simulink model "VOO"  (R2022a)
settings: Solver=FixedStepAuto  StartTime=0.0  StopTime=5  FixedStep=1e-3  RelTol=1e-3  EnableMultiTasking=on
undefined symbols (not defined in the file): D10, D11, D12, D2, D5, D8, D9, PTA0, PTA2, PTB9, PTC4, PTD0, PTD2, PTD3
libraries: frdmk64flib x8
settings Model: ExtModeTrigDuration=5  Creator=tygre  LastModifiedBy=tygre
settings OptimizationCC: EnhancedBackFolding=on  PassReuseOutputArgsAs=Individual arguments  ZeroExternalMemoryAtStartup=off  ZeroInternalMemoryAtStartup=off  MaxStackSize=64  OptimizeBlockOrder=speed  DifferentSizesBufferReuse=on  OptimizationCustomize=off  EfficientTunableParamExpr=on
settings DebuggingCC: ParameterTunabilityLossMsg=error
settings HardwareCC: ProdBitPerPointer=32  ProdBitPerSizeT=32  ProdBitPerPtrDiffT=32  ProdLargestAtomicInteger=Long  ProdLargestAtomicFloat=Double  ProdWordSize=32  ProdHWDeviceType=ARM Compatible->ARM Cortex
settings SFSimCC: MATLABDynamicMemAlloc=off
settings RTWCC: SystemTargetFile=ert.tlc  HardwareBoard=NXP FRDM-K64F  TLCOptions="-aInlineSetEventsForThisBaseRateFcn=TLC_FALSE -aSuppressMultiTaskScheduler=TLC_FALSE  -aRateBasedStepFcn=0"  TemplateMakefile=ert_default_tmf  Toolchain=GNU Tools for ARM Embedded Processors
settings CodeAppCC: ForceParamTrailComments=on  IgnoreCustomStorageClasses=off  OperatorAnnotations=on  SimulinkDataObjDesc=on  SFDataObjDesc=on  InsertBlockDesc=on
settings ERTTargetCC: ExtModeTransport=4  ExtModeMexFile=sendToCommService

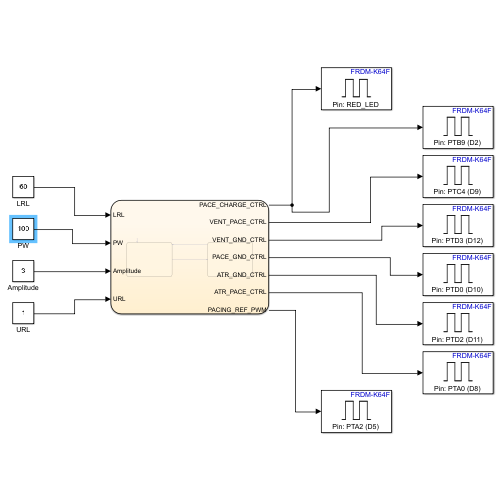
[thumbnail: Simulink's stored preview of the top-level diagram]
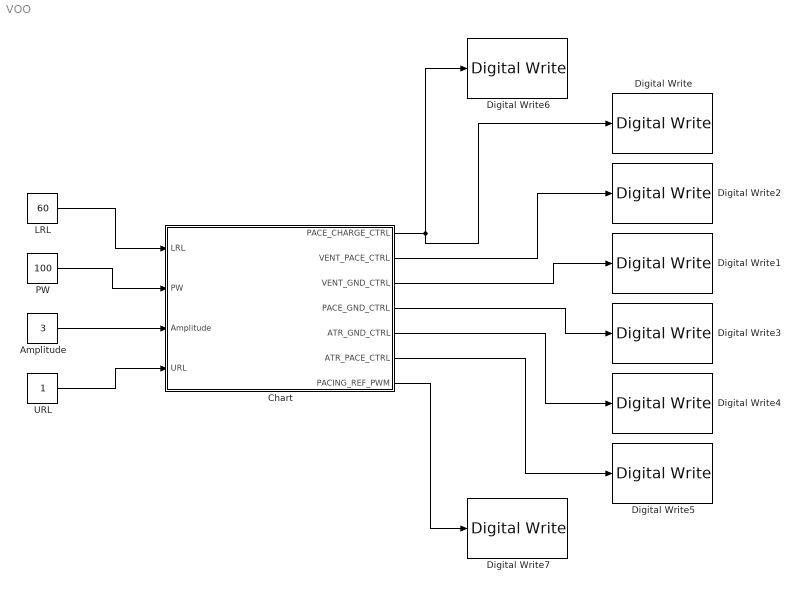
== system VOO ==
  Amplitude : Constant  Value=3  OutDataTypeStr=double
  Chart : Stateflow chart  TreatAsAtomicUnit=on
  Digital Write : frdmk64flib/Digital Write  Whichpin=PTB9 (D2)
  Digital Write1 : frdmk64flib/Digital Write  Whichpin=PTD3 (D12)
  Digital Write2 : frdmk64flib/Digital Write  Whichpin=PTC4 (D9)
  Digital Write3 : frdmk64flib/Digital Write  Whichpin=PTD0 (D10)
  Digital Write4 : frdmk64flib/Digital Write  Whichpin=PTD2 (D11)
  Digital Write5 : frdmk64flib/Digital Write  Whichpin=PTA0 (D8)
  Digital Write6 : frdmk64flib/Digital Write  Whichpin=RED_LED
  Digital Write7 : frdmk64flib/Digital Write  Whichpin=PTA2 (D5)
  LRL : Constant  Value=60
  PW : Constant  Value=100
  URL : Constant
  wires:
  LRL/1 -> Chart/1(LRL)
  PW/1 -> Chart/2(PW)
  Amplitude/1 -> Chart/3(Amplitude)
  URL/1 -> Chart/4(URL)
  Chart/1(PACE_CHARGE_CTRL) -> Digital Write/1, Digital Write6/1
  Chart/2(VENT_PACE_CTRL) -> Digital Write2/1
  Chart/3(VENT_GND_CTRL) -> Digital Write1/1
  Chart/4(PACE_GND_CTRL) -> Digital Write3/1
  Chart/5(ATR_GND_CTRL) -> Digital Write4/1
  Chart/6(ATR_PACE_CTRL) -> Digital Write5/1
  Chart/7(PACING_REF_PWM) -> Digital Write7/1

== stateflow chart VOO/Chart ==
  state C22_CHARGE
    entry:
    ATR_PACE_CTRL = false;
    VENT_PACE_CTRL = false;
    PACING_REF_PWM = (Amplitude / 5) *100;
    PACE_CHARGE_CTRL = true;
    PACE_GND_CTRL = true;
    ATR_GND_CTRL = false;
    VENT_GND_CTRL = true ;
  state C22_DISCHARGE
    entry:
    PACE_CHARGE_CTRL = false;
    PACE_GND_CTRL = true;
    ATR_PACE_CTRL = false;
    ATR_GND_CTRL = false;
    VENT_GND_CTRL = false;
    VENT_PACE_CTRL = true;
  (default) -> C22_CHARGE
  C22_DISCHARGE -> C22_CHARGE : after(PW,msec)
  C22_CHARGE -> C22_DISCHARGE : after(((60000/LRL)-PW),msec)
  data: PACE_CHARGE_CTRL output boolean; VENT_PACE_CTRL output boolean; VENT_GND_CTRL output boolean; PACE_GND_CTRL output boolean; LRL input double; PW input double; Amplitude input double; URL input double; ATR_GND_CTRL output boolean; ATR_PACE_CTRL output boolean; PACING_REF_PWM output double
